simulink model "sim_p"  (R2013b)
settings: Solver=ode45  StartTime=0.0  StopTime=10.0  RelTol=1e-3
libraries: commanapbnd3 x2
settings Model: Creator=Kseniya  LastModifiedBy=Kseniya

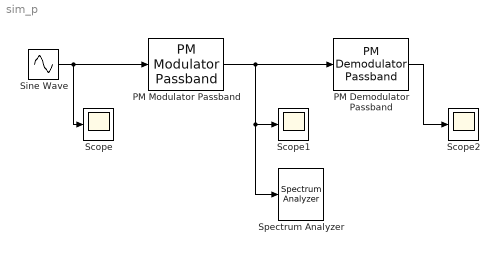
== system sim_p ==
  PM Demodulator Passband : commanapbnd3/PM Demodulator Passband  Fc=300  Ph=0  Kc=pi/2  Ho=100
  PM Modulator Passband : commanapbnd3/PM Modulator Passband  Fc=300  Ph=0  Kc=pi/2
  Scope : Scope
  Scope1 : Scope
      settings: TimeRange=0.2031838875481653  YMin=-2.5  YMax=0
  Scope2 : Scope
      settings: SaveName=ScopeData2
  Sine Wave : Sin  Amplitude=4  SampleTime=1/300
  Spectrum Analyzer : SpectrumAnalyzer
      settings: CopyFcn=scopeextensions.ScopeBlock.onCoreBlockCopy(gcbh);  DeleteFcn=scopeextensions.ScopeBlock.callback(gcbh, 'onBlockDelete');  PreSaveFcn=scopeextensions.ScopeBlock.callback(gcbh, 'onModelSave');  NameChangeFcn=scopeextensions.ScopeBlock.callback(gcbh, 'onBlockRename');  DestroyFcn=scopeextensions.ScopeBlock.onBlockDestroy(gcbh)  CloseFcn=scopeextensions.ScopeBlock.callback(gcbh, 'onBlockClose');  PreDeleteFcn=scopeextensions.ScopeBlock.callback(gcbh, 'onBlockPreDelete');
  wires:
  Sine Wave/1 -> PM Modulator Passband/1, Scope/1
  PM Modulator Passband/1 -> PM Demodulator Passband/1, Scope1/1, Spectrum Analyzer/1
  PM Demodulator Passband/1 -> Scope2/1
